simulink model "Q2_a1"  (R2015a)
settings: Solver=ode45  StartTime=0.0  StopTime=1  RelTol=1e-10  AbsTol=1e-10
libraries: cstblocks x4
settings Model: Creator=yarde_000  LastModifiedBy=yarde_000

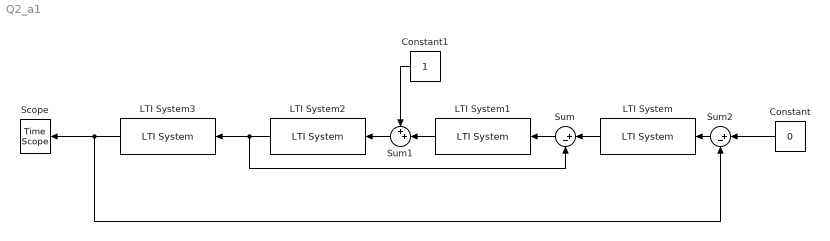
== system Q2_a1 ==
  Constant : Constant  Value=0
  Constant1 : Constant
  LTI System : cstblocks/LTI System  sys=Cp  IC=[]
  LTI System1 : cstblocks/LTI System  sys=Cpi  IC=[]
  LTI System2 : cstblocks/LTI System  sys=P  IC=[]
  LTI System3 : cstblocks/LTI System  sys=tf(1, [1 0])  IC=[]
  Scope : TimeScope
  Sum : Sum  Inputs=|+-
  Sum1 : Sum  Inputs=++|
  Sum2 : Sum  Inputs=|+-
  wires:
  Sum/1 -> LTI System1/1
  LTI System/1 -> Sum/1
  LTI System2/1 -> Sum/2, LTI System3/1
  Sum2/1 -> LTI System/1
  Constant/1 -> Sum2/1
  LTI System3/1 -> Scope/1, Sum2/2
  Sum1/1 -> LTI System2/1
  LTI System1/1 -> Sum1/2
  Constant1/1 -> Sum1/1
